simulink library "MOTH"  (R2016a)
settings: Solver=ode45  StartTime=0.0  StopTime=10.0  RelTol=1e-3
undefined symbols (not defined in the file): CAL_backwardErrorVal, CAL_ErrorLimit, CAL_ErrorLowerLimit, CAL_forwardErrorLimit, CAL_forwardStartIncr, CAL_MOTOR_HIGH, CAL_MOTOR_LOW, CONST_NegOne, CONST_noVelocity, ENU_BACKWARD, ENU_FORWARD, ENU_STOP
libraries: simulink x1
settings Model: Creator=oelkawok  LastModifiedBy=oelkawok
settings DataIOCC: LimitDataPoints=on
settings DebuggingCC: AllowSymbolicDim=off

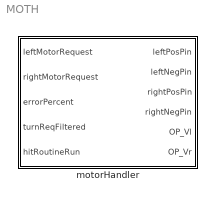
== system MOTH ==
  motorHandler : Subsystem

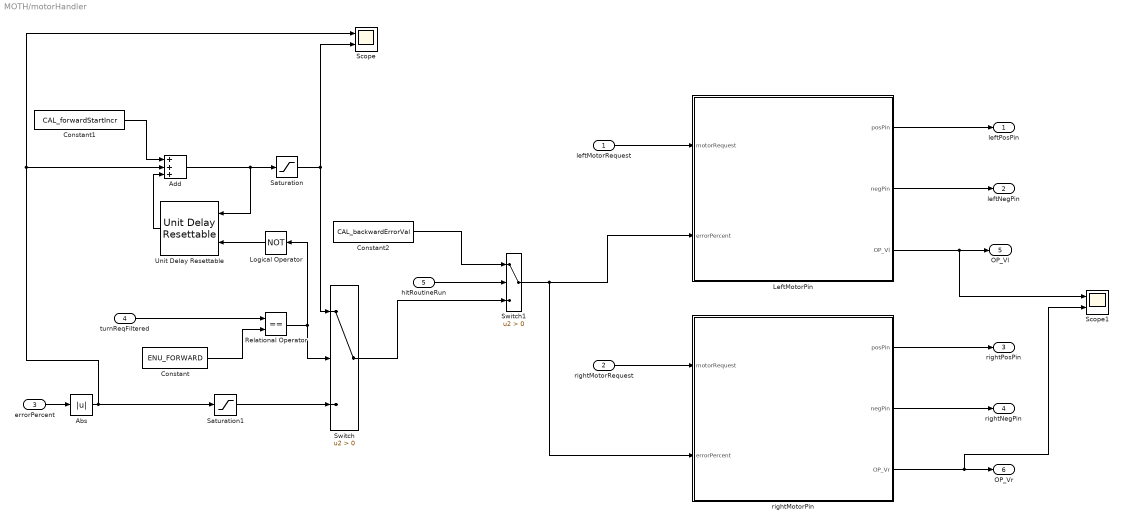
== system MOTH/motorHandler ==
  leftMotorRequest : Inport
  rightMotorRequest : Inport  Port=2
  errorPercent : Inport  Port=3
  turnReqFiltered : Inport  Port=4
  hitRoutineRun : Inport  Port=5
  Abs : Abs
  Add : Sum  Inputs=+++
  Constant : Constant  Value=ENU_FORWARD
  Constant1 : Constant  Value=CAL_forwardStartIncr
  Constant2 : Constant  Value=CAL_backwardErrorVal
  LeftMotorPin : Subsystem
  Logical Operator : Logic  Operator=NOT  AllPortsSameDT=off  OutDataTypeStr=boolean
  Relational Operator : RelationalOperator  Operator===  OutDataTypeStr=boolean
  Saturation : Saturate  UpperLimit=CAL_forwardErrorLimit  LowerLimit=0
      settings: AttributesFormatString=|
      | upper: %<UpperLimit>
      | Lower: %<LowerLimit>
  Saturation1 : Saturate  UpperLimit=CAL_ErrorLimit  LowerLimit=CAL_ErrorLowerLimit
      settings: AttributesFormatString=|
      | upper: %<UpperLimit>
      | lower: %<LowerLimit>
  Scope : Scope  NumInputPorts=2
  Scope1 : Scope  NumInputPorts=2
  Switch : Switch  Criteria=u2 > Threshold
  Switch1 : Switch  Criteria=u2 > Threshold
  Unit Delay Resettable : simulink/Additional Math & Discrete/Additional Discrete/Unit Delay Resettable  vinit=0.001  tsamp=-1
  rightMotorPin : Subsystem
  leftPosPin : Outport
  leftNegPin : Outport  Port=2
  rightPosPin : Outport  Port=3
  rightNegPin : Outport  Port=4
  OP_Vl : Outport  Port=5
  OP_Vr : Outport  Port=6
  wires:
  Switch1/1 -> LeftMotorPin/2(errorPercent), rightMotorPin/2(errorPercent)
  Constant2/1 -> Switch1/1
  hitRoutineRun/1 -> Switch1/2
  Switch/1 -> Switch1/3
  Saturation1/1 -> Switch/3
  Logical Operator/1 -> Unit Delay Resettable/2
  Constant1/1 -> Add/1
  Relational Operator/1 -> Switch/2, Logical Operator/1
  Saturation/1 -> Scope/2, Switch/1
  Add/1 -> Saturation/1, Unit Delay Resettable/1
  Unit Delay Resettable/1 -> Add/3
  Abs/1 -> Saturation1/1, Scope/1, Add/2
  Constant/1 -> Relational Operator/2
  turnReqFiltered/1 -> Relational Operator/1
  errorPercent/1 -> Abs/1
  rightMotorRequest/1 -> rightMotorPin/1(motorRequest)
  rightMotorPin/2(negPin) -> rightNegPin/1
  rightMotorPin/1(posPin) -> rightPosPin/1
  LeftMotorPin/2(negPin) -> leftNegPin/1
  LeftMotorPin/1(posPin) -> leftPosPin/1
  leftMotorRequest/1 -> LeftMotorPin/1(motorRequest)
  LeftMotorPin/3(OP_Vl) -> OP_Vl/1, Scope1/1
  rightMotorPin/3(OP_Vr) -> OP_Vr/1, Scope1/2

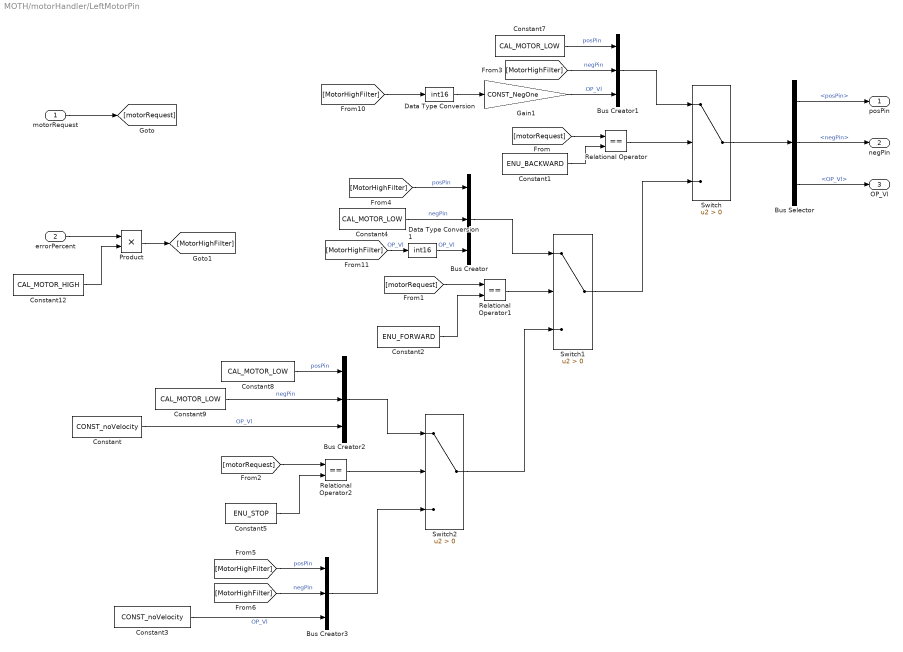
== system MOTH/motorHandler/LeftMotorPin ==
  motorRequest : Inport
  errorPercent : Inport  Port=2
  Bus Creator{,1..3} (4 alike) : BusCreator  Inputs=3
  Bus Selector : BusSelector  OutputSignals=posPin,negPin,OP_Vl
  Constant : Constant  Value=CONST_noVelocity
  Constant1 : Constant  Value=ENU_BACKWARD
  Constant12 : Constant  Value=CAL_MOTOR_HIGH
  Constant2 : Constant  Value=ENU_FORWARD
  Constant3 : Constant  Value=CONST_noVelocity
  Constant{4,7..9} (4 alike) : Constant  Value=CAL_MOTOR_LOW
  Constant5 : Constant  Value=ENU_STOP
  Data Type Conversion : DataTypeConversion  OutDataTypeStr=int16
  Data Type Conversion1 : DataTypeConversion  OutDataTypeStr=int16
  Gain1 : Gain  Gain=CONST_NegOne  OutDataTypeStr=int8
  Product : Product  OutDataTypeStr=uint8
  Relational Operator : RelationalOperator  Operator===  OutDataTypeStr=boolean
  Relational Operator1 : RelationalOperator  Operator===  OutDataTypeStr=boolean
  Relational Operator2 : RelationalOperator  Operator===  OutDataTypeStr=boolean
  Switch : Switch  Criteria=u2 > Threshold
  Switch1 : Switch  Criteria=u2 > Threshold
  Switch2 : Switch  Criteria=u2 > Threshold
  posPin : Outport
  negPin : Outport  Port=2
  OP_Vl : Outport  Port=3
  wires:
  Data Type Conversion1/1 -> Bus Creator/3  "OP_Vl"
  Data Type Conversion/1 -> Gain1/1
  Bus Selector/3 -> OP_Vl/1  "<OP_Vl>"
  Constant3/1 -> Bus Creator3/3  "OP_Vl"
  Constant/1 -> Bus Creator2/3  "OP_Vl"
  [MotorHighFilter] -> Data Type Conversion1/1  "OP_Vl"
  Gain1/1 -> Bus Creator1/3  "OP_Vl"
  [MotorHighFilter] -> Data Type Conversion/1
  Bus Selector/2 -> negPin/1  "<negPin>"
  Bus Selector/1 -> posPin/1  "<posPin>"
  Switch/1 -> Bus Selector/1
  [motorRequest] -> Relational Operator1/1
  [motorRequest] -> Relational Operator/1
  motorRequest/1 -> [motorRequest]
  Bus Creator3/1 -> Switch2/3
  Switch2/1 -> Switch1/3
  [MotorHighFilter] -> Bus Creator3/1  "posPin"
  Constant9/1 -> Bus Creator2/2  "negPin"
  Relational Operator2/1 -> Switch2/2
  [MotorHighFilter] -> Bus Creator3/2  "negPin"
  [motorRequest] -> Relational Operator2/1
  Bus Creator1/1 -> Switch/1
  Bus Creator2/1 -> Switch2/1
  Bus Creator/1 -> Switch1/1
  Constant8/1 -> Bus Creator2/1  "posPin"
  Switch1/1 -> Switch/3
  Constant7/1 -> Bus Creator1/1  "posPin"
  Constant5/1 -> Relational Operator2/2
  Constant2/1 -> Relational Operator1/2
  Relational Operator/1 -> Switch/2
  Constant1/1 -> Relational Operator/2
  [MotorHighFilter] -> Bus Creator1/2  "negPin"
  [MotorHighFilter] -> Bus Creator/1  "posPin"
  Constant4/1 -> Bus Creator/2  "negPin"
  Relational Operator1/1 -> Switch1/2
  errorPercent/1 -> Product/1
  Constant12/1 -> Product/2
  Product/1 -> [MotorHighFilter]

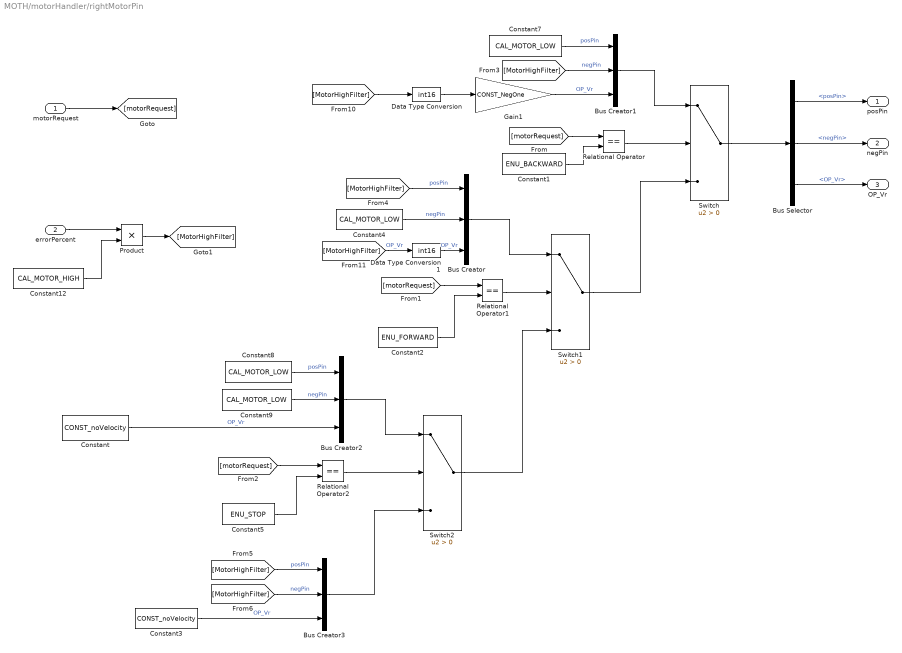
== system MOTH/motorHandler/rightMotorPin ==
  motorRequest : Inport
  errorPercent : Inport  Port=2
  Bus Creator{,1..3} (4 alike) : BusCreator  Inputs=3
  Bus Selector : BusSelector  OutputSignals=posPin,negPin,OP_Vr
  Constant : Constant  Value=CONST_noVelocity
  Constant1 : Constant  Value=ENU_BACKWARD
  Constant12 : Constant  Value=CAL_MOTOR_HIGH
  Constant2 : Constant  Value=ENU_FORWARD
  Constant3 : Constant  Value=CONST_noVelocity
  Constant{4,7..9} (4 alike) : Constant  Value=CAL_MOTOR_LOW
  Constant5 : Constant  Value=ENU_STOP
  Data Type Conversion : DataTypeConversion  OutDataTypeStr=int16
  Data Type Conversion1 : DataTypeConversion  OutDataTypeStr=int16
  Gain1 : Gain  Gain=CONST_NegOne  OutDataTypeStr=int8
  Product : Product  OutDataTypeStr=uint8
  Relational Operator : RelationalOperator  Operator===  OutDataTypeStr=boolean
  Relational Operator1 : RelationalOperator  Operator===  OutDataTypeStr=boolean
  Relational Operator2 : RelationalOperator  Operator===  OutDataTypeStr=boolean
  Switch : Switch  Criteria=u2 > Threshold
  Switch1 : Switch  Criteria=u2 > Threshold
  Switch2 : Switch  Criteria=u2 > Threshold
  posPin : Outport
  negPin : Outport  Port=2
  OP_Vr : Outport  Port=3
  wires:
  Data Type Conversion1/1 -> Bus Creator/3  "OP_Vr"
  Data Type Conversion/1 -> Gain1/1
  Product/1 -> [MotorHighFilter]
  Constant12/1 -> Product/2
  errorPercent/1 -> Product/1
  Relational Operator1/1 -> Switch1/2
  Constant4/1 -> Bus Creator/2  "negPin"
  [MotorHighFilter] -> Bus Creator/1  "posPin"
  [MotorHighFilter] -> Bus Creator1/2  "negPin"
  Constant1/1 -> Relational Operator/2
  Relational Operator/1 -> Switch/2
  Constant2/1 -> Relational Operator1/2
  Constant5/1 -> Relational Operator2/2
  Constant7/1 -> Bus Creator1/1  "posPin"
  Switch1/1 -> Switch/3
  Constant8/1 -> Bus Creator2/1  "posPin"
  Bus Creator/1 -> Switch1/1
  Bus Creator2/1 -> Switch2/1
  Bus Creator1/1 -> Switch/1
  [motorRequest] -> Relational Operator2/1
  [MotorHighFilter] -> Bus Creator3/2  "negPin"
  Relational Operator2/1 -> Switch2/2
  Constant9/1 -> Bus Creator2/2  "negPin"
  [MotorHighFilter] -> Bus Creator3/1  "posPin"
  Switch2/1 -> Switch1/3
  Bus Creator3/1 -> Switch2/3
  motorRequest/1 -> [motorRequest]
  [motorRequest] -> Relational Operator/1
  [motorRequest] -> Relational Operator1/1
  Switch/1 -> Bus Selector/1
  Bus Selector/1 -> posPin/1  "<posPin>"
  Bus Selector/2 -> negPin/1  "<negPin>"
  [MotorHighFilter] -> Data Type Conversion/1
  Gain1/1 -> Bus Creator1/3  "OP_Vr"
  [MotorHighFilter] -> Data Type Conversion1/1  "OP_Vr"
  Constant/1 -> Bus Creator2/3  "OP_Vr"
  Constant3/1 -> Bus Creator3/3  "OP_Vr"
  Bus Selector/3 -> OP_Vr/1  "<OP_Vr>"
